simulink model "brayton_cycle_LSTM_ROM"  (R2023a)
settings: Solver=ode23t  StartTime=0.0  StopTime=1000  RelTol=1e-3
PreLoadFcn:
  | combustor_volume = 0.001; % m^3
  | flow_area = 0.002; % m^2;
  | shaft_inertia = 0.1; % kg*m^2
  | mechanical_efficiency = 0.98; % 1
  | apu_shaft_speed = 6000; % rpm
  | 
  | % Compressor Map
  | 
  | compressor.beta_vector = [
  |      0, 0.1, 0.2, 0.3, 0.4, 0.5, 0.6, 0.7, 0.8, 0.9, 1.0];
  | 
  | compressor.corrected_speed_vector = [
  |     5000, 6000, 7000, 8000, 8500, 9000, 9500, 10000, 11000, 12000
  |     ]; % rpm
  | 
  | compressor.map.pressure_ratio = [
  |     0.1806    0.4817    0.8258    1.1561    1.4451    1.7002    2.0645    2.4086    2.6275    2.7527    2.8903
  |     0.2364    0.6303    1.0806    1.5128    1.8910    2.2247    2.7014    3.1517    3.4382    3.6019    3.7820
  |     0.2921    0.7790    1.3354    1.8695    2.3369    2.7493    3.3384    3.8948    4.2489    4.4512    4.6738
  |     0.4031    1.0748    1.8425    2.5795    3.2244    3.7934    4.6063    5.3740    5.8625    6.1417    6.4488
  |     0.5503    1.4673    2.5155    3.5216    4.4021    5.1789    6.2886    7.3368    8.0037    8.3849    8.8041
  |     0.7404    1.9745    3.3849    4.7388    5.9235    6.9688    8.4621    9.8725   10.7700   11.2829   11.8470
  |     0.9903    2.6407    4.5270    6.3378    7.9222    9.3203   11.3175   13.2037   14.4041   15.0900   15.8445
  |     1.2261    3.2697    5.6051    7.8472    9.8090   11.5400   14.0129   16.3483   17.8345   18.6838   19.6180
  |     1.2827    3.4206    5.8639    8.2094   10.2617   12.0726   14.6596   17.1029   18.6577   19.5462   20.5235
  |     1.3393    3.5715    6.1226    8.5716   10.7145   12.6053   15.3064   17.8575   19.4809   20.4086   21.4290]; % 1
  | 
  | compressor.map.corrected_mass_flow_rate = [
  |     0.0400    0.0400    0.0400    0.0399    0.0395    0.0389    0.0378    0.0363    0.0349    0.0340    0.0329
  |     0.0530    0.0530    0.0530    0.0527    0.0521    0.0513    0.0501    0.0481    0.0462    0.0449    0.0434
  |     0.0640    0.0640    0.0639    0.0635    0.0630    0.0623    0.0611    0.0589    0.0565    0.0549    0.0530
  |     0.1000    0.1000    0.0997    0.0991    0.0983    0.0974    0.0951    0.0906    0.0870    0.0846    0.0814
  |     0.1350    0.1350    0.1346    0.1340    0.1332    0.1324    0.1301    0.1258    0.1222    0.1197    0.1165
  |     0.1700    0.1699    0.1695    0.1688    0.1681    0.1673    0.1654    0.1620    0.1589    0.1562    0.1521
  |     0.2100    0.2097    0.2089    0.2077    0.2064    0.2051    0.2021    0.1978    0.1925    0.1882    0.1824
  |     0.2500    0.2498    0.2494    0.2488    0.2480    0.2472    0.2452    0.2414    0.2375    0.2338    0.2287
  |     0.2600    0.2599    0.2595    0.2589    0.2581    0.2574    0.2555    0.2516    0.2482    0.2453    0.2415
  |     0.2640    0.2639    0.2635    0.2629    0.2622    0.2616    0.2604    0.2580    0.2558    0.2542    0.2513]; % kg/s
  | 
  | compressor.map.efficiency = [
  |     0.3500    0.4200    0.4900    0.5600    0.5950    0.6300    0.6650    0.6860    0.6650    0.5600    0.4900
  |     0.3600    0.4320    0.5040    0.5760    0.6120    0.6480    0.6840    0.7056    0.6840    0.5760    0.5040
  |     0.3750    0.4500    0.5250    0.6000    0.6375    0.6750    0.7125    0.7350    0.7125    0.6000    0.5250
  |     0.3900    0.4680    0.5460    0.6240    0.6630    0.7020    0.7410    0.7644    0.7410    0.6240    0.5460
  |     0.4000    0.4800    0.5600    0.6400    0.6800    0.7200    0.7600    0.7840    0.7600    0.6400    0.5600
  |     0.4250    0.5100    0.5950    0.6800    0.7225    0.7650    0.8075    0.8330    0.8075    0.6800    0.5950
  |     0.4500    0.5400    0.6300    0.7200    0.7650    0.8100    0.8550    0.8820    0.8550    0.7200    0.6300
  |     0.4900    0.5880    0.6860    0.7840    0.8330    0.8820    0.9310    0.9604    0.9310    0.7840    0.6860
  |     0.4500    0.5400    0.6300    0.7200    0.7650    0.8100    0.8550    0.8820    0.8550    0.7200    0.6300
  |     0.4000    0.4800    0.5600    0.6400    0.6800    0.7200    0.7600    0.7840    0.7600    0.6400    0.5600]; % 1
  | 
  | compressor.reference_pressure = 0.101325; % MPa
  | compressor.reference_temperature = 288.15; % K
  | 
  | % Turbine Map
  | 
  | turbine.flow_map.pressure_ratio = [
  |     1.0010, 1.0050, 1.0101, 1.0204, 1.0309, 1.0417, 1.0526, 1.1111, 1.1765, 1.2500, 1.3333, 1.4286, 1.5385, 1.6667, 1.8182, 2.0000
  |     ]; %  1
  | turbine.flow_map.corrected_mass_flow_rate = [
  |     0.0523, 0.1168, 0.1647, 0.2316, 0.2822, 0.3240, 0.3601, 0.4945, 0.5871, 0.6560, 0.7079, 0.7465, 0.7739, 0.7912, 0.7993, 0.8000
  |     ]; % kg/s
  | 
  | turbine.efficiency_map.pressure_ratio = [1.1111, 1.2500, 1.4286, 1.6667, 2.0000, 2.5000, 3.3333, 5.0000];
  | turbine.efficiency_map.isentropic_efficiency = [0.7500, 0.8100, 0.8400, 0.8500, 0.8500, 0.8450, 0.8300, 0.8000];
  | 
  | turbine.reference_pressure = 1.5; % MPa
  | turbine.reference_temperature = 1000; % K
  | 
  | % APU Map
  | 
  | apu = turbine;
  | apu.reference_pressure = 0.5; % MPa
  | apu.reference_temperature = 600; % K
  | 
  | % Set Scale Factor
  | scale_factor = 1;
model workspace (MAT data in the model file):
  RPM_refMean = 7784.53870936
  RPM_refStd = 2217.44936474
  initT3 = 288.15
  normFactor = 1000
  phiMean = 95.1498183593
  phiStd = 99.1536281541
  powerMean = 39.0528228451
  powerStd = 37.5156635245
  rpm0 = 4500
  rpmMean = 7778.84746986
  rpmStd = 2213.65213434
  rpm_setpoint = [4000 4000 5000 5000 6000 6000 7000 7000 8000 8000 9000 9000 10000 10000 11000 11000 12000 12000 12000]
  samplTime = 0.1
  t3Mean = 1034.93127137
  t3Std = 345.320803836
  time_setpoint = [0 200 220 300 320 400 420 500 520 600 620 700 720 800 820 900 920 1000 1100]
undefined symbols (not defined in the file): scenario
libraries: deeplib x1, simulink x1
CloseFcn:
  | try,close(h1_sscfluids_brayton_cycle),end
  | clear h1_sscfluids_brayton_cycle
  | try,close(h2_sscfluids_brayton_cycle),end
  | clear h2_sscfluids_brayton_cycle
  | try,close(h3_sscfluids_brayton_cycle),end
  | clear h3_sscfluids_brayton_cycle
  | try,close(h4_sscfluids_brayton_cycle),end
  | clear h4_sscfluids_brayton_cycle
  | 
  | clear combustor_volume flow_area shaft_inertia mechanical_efficiency apu_shaft_speed
  | clear compressor turbine apu
  | clear simlog_sscfluids_brayton_cycle tout
  | clear scale_factor user_input
Description:
  | Brayton Cycle (Gas Turbine)
settings Model: Creator=The MathWorks, Inc.  LastModifiedBy=imyrsini
settings SolverCC: MaxConsecutiveMinStep=2  AlgebraicLoopSolver=TrustRegion
settings DataIOCC: ReturnWorkspaceOutputs=off
settings OptimizationCC: DefaultParameterBehavior=Inlined  EnhancedBackFolding=on  PassReuseOutputArgsAs=Individual arguments  ZeroExternalMemoryAtStartup=off  ZeroInternalMemoryAtStartup=off  OptimizeBlockOrder=speed  DifferentSizesBufferReuse=on  OptimizationCustomize=off  EfficientTunableParamExpr=on
settings DebuggingCC: ParameterTunabilityLossMsg=error  UnconnectedInputMsg=warning  UnconnectedOutputMsg=warning  UnconnectedLineMsg=warning  PregeneratedLibrarySubsystemCodeDiagnostic=none  ArithmeticOperatorsInVariantConditions=warning
settings ModelReferenceCC: EnableRefExpFcnMdlSchedulingChecks=on
settings SFSimCC: SimUseLocalCustomCode=off  MATLABDynamicMemAlloc=off  CustomCodeUndefinedFunction=UseInterfaceOnly
settings RTWCC: Description=Embedded Coder  SystemTargetFile=ert.tlc  TemplateMakefile=ert_default_tmf  RTWUseLocalCustomCode=off  DLArmComputeVersion=19.05
settings CodeAppCC: ForceParamTrailComments=on  IgnoreCustomStorageClasses=off  OperatorAnnotations=on  SimulinkDataObjDesc=on  SFDataObjDesc=on  InsertBlockDesc=on
settings ERTTargetCC: TargetLangStandard=C99 (ISO)  GenerateSampleERTMain=on  InlinedParameterPlacement=NonHierarchical  ERTCustomFileTemplate=example_file_process.tlc
settings SimscapeCC: SimscapeLogType=all  SimscapeLogSimulationStatistics=on  SimscapeLogName=simlog_sscfluids_brayton_cycle  SimscapeLogDataHistory=10000

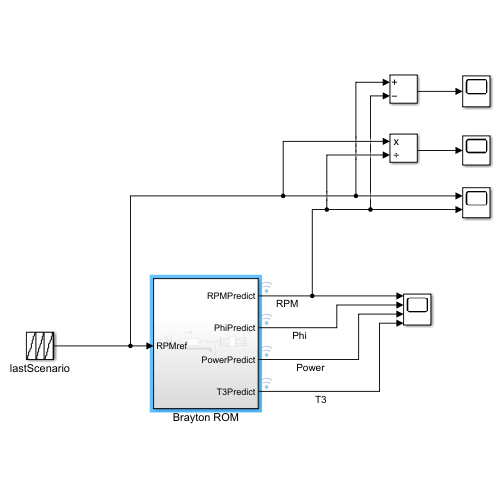
[thumbnail: Simulink's stored preview of the top-level diagram]
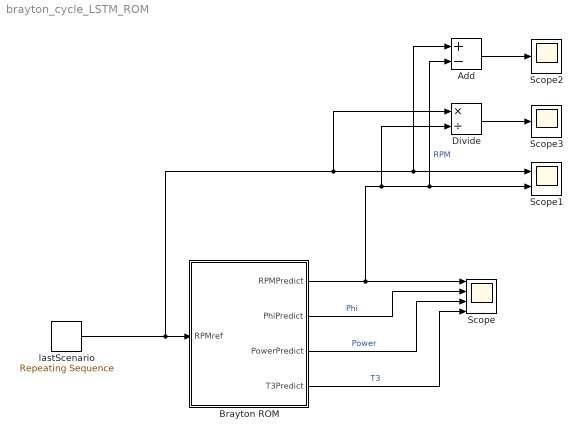
== system brayton_cycle_LSTM_ROM ==
  Add : Sum  Inputs=+-
  Brayton ROM : Subsystem
  Divide : Product  Inputs=*/
  Scope : Scope  NumInputPorts=4
  Scope1 : Scope  NumInputPorts=2
  Scope2 : Scope
  Scope3 : Scope
  lastScenario : simulink/Sources/Repeating Sequence  rep_seq_t=scenario{6}.shaftSpeedRef{1}.Values.Time'  rep_seq_y=scenario{6}.shaftSpeedRef{1}.Values.Data'
  wires:
  lastScenario/1 -> Divide/1, Add/1, Scope1/1, Brayton ROM/1(RPMref)
  Brayton ROM/1(RPMPredict) -> Divide/2, Add/2, Scope1/2, Scope/1  "RPM"
  Brayton ROM/2(PhiPredict) -> Scope/2  "Phi"
  Brayton ROM/3(PowerPredict) -> Scope/3  "Power"
  Brayton ROM/4(T3Predict) -> Scope/4  "T3"
  Add/1 -> Scope2/1
  Divide/1 -> Scope3/1

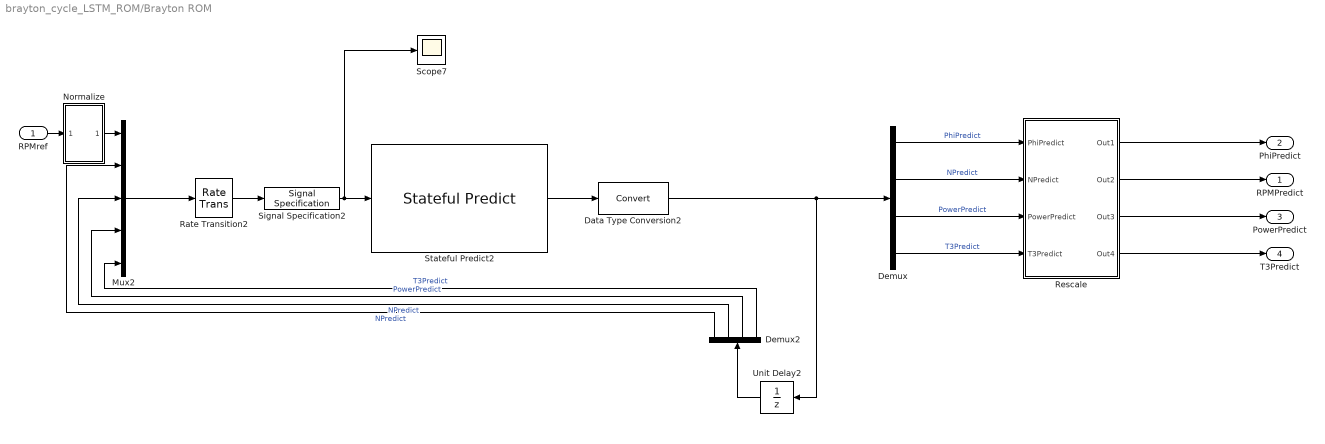
== system brayton_cycle_LSTM_ROM/Brayton ROM ==
  RPMref : Inport
  Data Type Conversion2 : DataTypeConversion  SaturateOnIntegerOverflow=off  RndMeth=Floor
  Demux : Demux
  Demux2 : Demux
  Mux2 : Mux  Inputs=5
  Normalize : Subsystem
  Rate Transition2 : RateTransition  OutPortSampleTime=samplTime
  Rescale : Subsystem
  Scope7 : Scope
  Signal Specification2 : SignalSpecification  Dimensions=[5 1]
  Stateful Predict2 : deeplib/Stateful Predict  Network=Network from MAT-file  NetworkFunction=untitled  NetworkFilePath=C:\Users\imyrsini\OneDrive - MathWorks\Documents\Projects\AEprojects\LSTM Model Reduction\BraytonGasTurbSimplified_LSTMReductionTrial\braytonLSTMNetThermoNorm.mat  InputDataFormats={'',''}  SampleTime=-1  ForceInterpretedSim=off  EnableDLNetwork=on
  Unit Delay2 : UnitDelay  InitialCondition=[0; (rpm0-rpmMean)/rpmStd; 0; (initT3-t3Mean)/t3Std]  SampleTime=-1  HasFrameUpgradeWarning=on
  RPMPredict : Outport
  PhiPredict : Outport  Port=2
  PowerPredict : Outport  Port=3
  T3Predict : Outport  Port=4
  wires:
  Demux2/3 -> Mux2/4  "PowerPredict"
  Stateful Predict2/1 -> Data Type Conversion2/1
  Rate Transition2/1 -> Signal Specification2/1
  Demux2/4 -> Mux2/5  "T3Predict"
  Unit Delay2/1 -> Demux2/1
  Demux2/2 -> Mux2/3  "NPredict"
  Signal Specification2/1 -> Stateful Predict2/1, Scope7/1
  Demux2/1 -> Mux2/2  "NPredict"
  Demux/1 -> Rescale/1(PhiPredict)  "PhiPredict"
  Demux/2 -> Rescale/2(NPredict)  "NPredict"
  Demux/3 -> Rescale/3(PowerPredict)  "PowerPredict"
  Demux/4 -> Rescale/4(T3Predict)  "T3Predict"
  Rescale/1(Out1) -> PhiPredict/1
  Rescale/2(Out2) -> RPMPredict/1
  Rescale/3(Out3) -> PowerPredict/1
  Rescale/4(Out4) -> T3Predict/1
  Data Type Conversion2/1 -> Unit Delay2/1, Demux/1
  Mux2/1 -> Rate Transition2/1
  RPMref/1 -> Normalize/1(In1)
  Normalize/1(Out1) -> Mux2/1

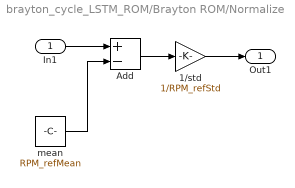
== system brayton_cycle_LSTM_ROM/Brayton ROM/Normalize ==
  In1 : Inport
  1/std : Gain  Gain=1/RPM_refStd
  Add : Sum  Inputs=+-
  mean : Constant  Value=RPM_refMean
  Out1 : Outport
  wires:
  In1/1 -> Add/1
  Add/1 -> 1/std/1
  mean/1 -> Add/2
  1/std/1 -> Out1/1

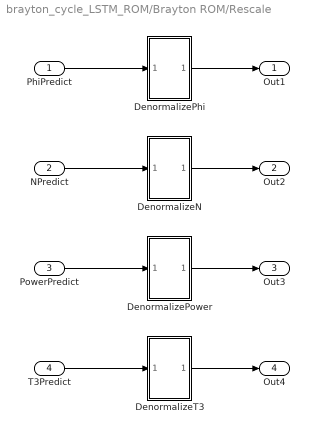
== system brayton_cycle_LSTM_ROM/Brayton ROM/Rescale ==
  PhiPredict : Inport
  NPredict : Inport  Port=2
  PowerPredict : Inport  Port=3
  T3Predict : Inport  Port=4
  DenormalizeN : Subsystem
  DenormalizePhi : Subsystem
  DenormalizePower : Subsystem
  DenormalizeT3 : Subsystem
  Out1 : Outport
  Out2 : Outport  Port=2
  Out3 : Outport  Port=3
  Out4 : Outport  Port=4
  wires:
  NPredict/1 -> DenormalizeN/1(NPredict)
  T3Predict/1 -> DenormalizeT3/1(T3Predict)
  PowerPredict/1 -> DenormalizePower/1(PowerPredict)
  PhiPredict/1 -> DenormalizePhi/1(PhiPredict)
  DenormalizePhi/1(Out1) -> Out1/1
  DenormalizeN/1(Out1) -> Out2/1
  DenormalizePower/1(Out1) -> Out3/1
  DenormalizeT3/1(Out1) -> Out4/1

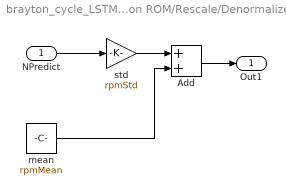
== system brayton_cycle_LSTM_ROM/Brayton ROM/Rescale/DenormalizeN ==
  NPredict : Inport
  Add : Sum
  mean : Constant  Value=rpmMean
  std : Gain  Gain=rpmStd
  Out1 : Outport
  wires:
  Add/1 -> Out1/1
  std/1 -> Add/1
  mean/1 -> Add/2
  NPredict/1 -> std/1

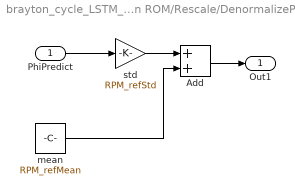
== system brayton_cycle_LSTM_ROM/Brayton ROM/Rescale/DenormalizePhi ==
  PhiPredict : Inport
  Add : Sum
  mean : Constant  Value=RPM_refMean
  std : Gain  Gain=RPM_refStd
  Out1 : Outport
  wires:
  PhiPredict/1 -> std/1
  mean/1 -> Add/2
  std/1 -> Add/1
  Add/1 -> Out1/1

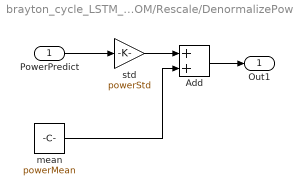
== system brayton_cycle_LSTM_ROM/Brayton ROM/Rescale/DenormalizePower ==
  PowerPredict : Inport
  Add : Sum
  mean : Constant  Value=powerMean
  std : Gain  Gain=powerStd
  Out1 : Outport
  wires:
  PowerPredict/1 -> std/1
  mean/1 -> Add/2
  std/1 -> Add/1
  Add/1 -> Out1/1

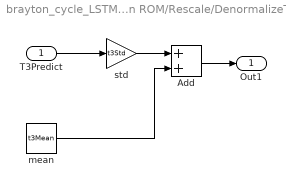
== system brayton_cycle_LSTM_ROM/Brayton ROM/Rescale/DenormalizeT3 ==
  T3Predict : Inport
  Add : Sum
  mean : Constant  Value=t3Mean
  std : Gain  Gain=t3Std
  Out1 : Outport
  wires:
  Add/1 -> Out1/1
  std/1 -> Add/1
  mean/1 -> Add/2
  T3Predict/1 -> std/1
